simulink model "Wing_Aero"  (R2023b)
settings: Solver=ode3  StartTime=0.0  StopTime=1  FixedStep=0.01  RelTol=1e-3
undefined symbols (not defined in the file): alpha_C_d, alpha_C_l, b_Wing_Half, c, C_d, C_l, dr, l_Wing, num_Blade, r, thickness_Wing, throttle, V
libraries: spsMeanLib x7, simulink_extras x2, matrix_library x1
settings Model: Creator=iwl  LastModifiedBy=iwl

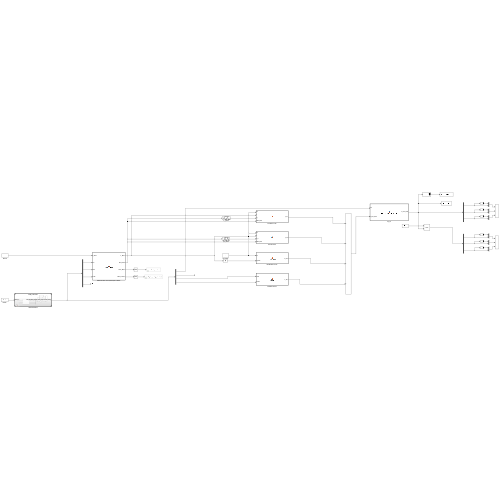
[thumbnail: Simulink's stored preview of the top-level diagram]
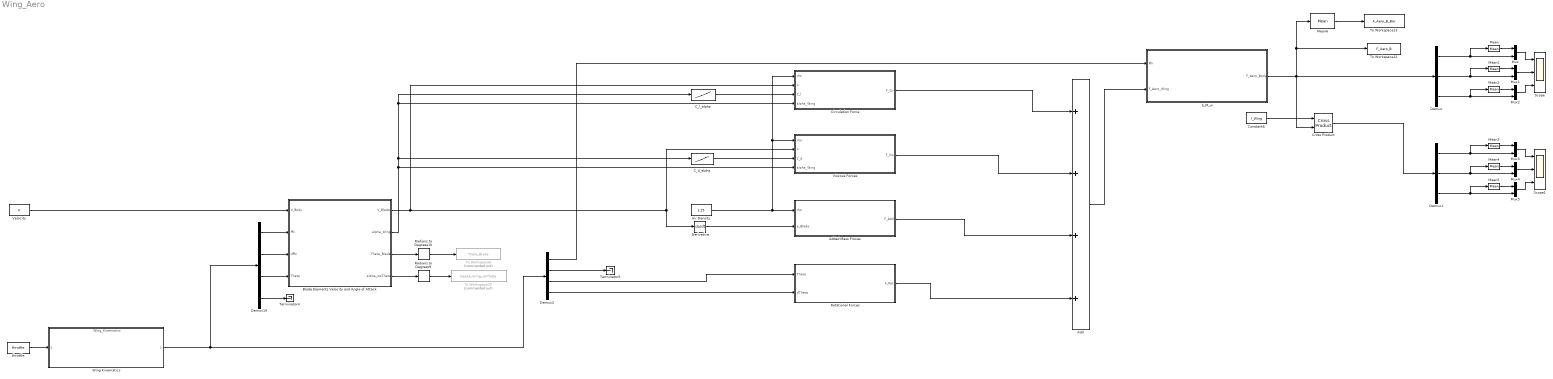
== system Wing_Aero ==
  Add : Sum  Inputs=++++
  Added Mass Froces : MATLAB Function  TreatAsAtomicUnit=on
  Air Density : Constant  Value=1.25
  Blade Elements Velocity and Angle of Attack : MATLAB Function  TreatAsAtomicUnit=on
  C_d_alpha : Lookup_n-D  NumberOfTableDimensions=1  BreakpointsForDimension1=alpha_C_d  Table=C_d  InternalRulePriority=Speed  RndMeth=Simplest
  C_l_alpha : Lookup_n-D  NumberOfTableDimensions=1  BreakpointsForDimension1=alpha_C_l  Table=C_l  InternalRulePriority=Speed  RndMeth=Simplest
  Circulation Force : MATLAB Function  TreatAsAtomicUnit=on
  Constant6 : Constant  Value=l_Wing
  Cross Product : matrix_library/Cross Product
  Demux : Demux  Outputs=3
  Demux1 : Demux  Outputs=3
  Demux19 : Demux
  Demux2 : Demux
  Derivative : Derivative
  Mean{,1..6} (7 alike) : spsMeanLib/Mean  Freq=f_max  Vinit=0  Ts=0
  Mux{,1..5} (6 alike) : Mux  Inputs=2
  Radians to Degrees10 : simulink_extras/Transformations/Radians to Degrees
  Radians to Degrees9 : simulink_extras/Transformations/Radians to Degrees
  Rotational Forces : MATLAB Function  TreatAsAtomicUnit=on
  Scope : Scope  NumInputPorts=3
  Scope1 : Scope  NumInputPorts=3
  Terminator4 : Terminator
  Terminator5 : Terminator
  To Workspace12 : ToWorkspace  VariableName=F_Aero_B  SampleTime=-1
  To Workspace13 : ToWorkspace  VariableName=F_Aero_B_Bar  SampleTime=-1
  To Workspace23 : ToWorkspace  Commented=on  VariableName=alapha_Wing_woTheta  SampleTime=-1
  To Workspace6 : ToWorkspace  Commented=on  VariableName=Theta_Blade  SampleTime=-1
  Velocity : Constant  Value=V
  Viscous Forces : MATLAB Function  TreatAsAtomicUnit=on
  Wing Kinematics : ModelReference  ModelNameDialog=Wing_Kinematics.slx  SimulationMode=Normal  ModelReferenceVersion=4.4
  b_M_w : MATLAB Function  TreatAsAtomicUnit=on
  throttle : Constant  Value=throttle
  wires:
  Demux19/4 -> Terminator4/1
  Radians to Degrees9/1 -> To Workspace23/1
  Demux2/2 -> Terminator5/1
  Demux19/1 -> Blade Elements Velocity and Angle of Attack/2(Phi)
  Blade Elements Velocity and Angle of Attack/3(Theta_Blade) -> Radians to Degrees10/1
  throttle/1 -> Wing Kinematics/1
  Demux19/2 -> Blade Elements Velocity and Angle of Attack/3(dPhi)
  Demux19/3 -> Blade Elements Velocity and Angle of Attack/4(Theta)
  Radians to Degrees10/1 -> To Workspace6/1
  Blade Elements Velocity and Angle of Attack/4(alpha_woTheta) -> Radians to Degrees9/1
  Wing Kinematics/1 -> Demux2/1, Demux19/1
  b_M_w/1(F_Aero_Body) -> Cross Product/2, Demux/1, Mean6/1, To Workspace12/1
  Add/1 -> b_M_w/2(F_Aero_Wing)
  Demux2/4 -> Rotational Forces/2(dTheta)
  Added Mass Froces/1(F_Add) -> Add/3
  Derivative/1 -> Added Mass Froces/2(a_Blade)
  Blade Elements Velocity and Angle of Attack/2(alpha_Wing) -> Circulation Force/4(alpha_Wing), C_l_alpha/1, C_d_alpha/1, Viscous Forces/4(alpha_Wing)
  C_l_alpha/1 -> Circulation Force/3(C_l)
  Circulation Force/1(F_Cir) -> Add/1
  Air Density/1 -> Circulation Force/1(rho), Viscous Forces/1(rho), Added Mass Froces/1(rho)
  Rotational Forces/1(F_Rot) -> Add/4
  Viscous Forces/1(F_Vis) -> Add/2
  C_d_alpha/1 -> Viscous Forces/3(C_d)
  Blade Elements Velocity and Angle of Attack/1(V_Blade) -> Viscous Forces/2(V), Derivative/1, Circulation Force/2(V)
  Constant6/1 -> Cross Product/1
  Demux2/1 -> b_M_w/1(Phi)
  Mean6/1 -> To Workspace13/1
  Demux2/3 -> Rotational Forces/1(Theta)
  Velocity/1 -> Blade Elements Velocity and Angle of Attack/1(V_Body)
  Demux/2 -> Mean1/1, Mux1/2
  Demux/1 -> Mux/2, Mean/1
  Demux/3 -> Mean2/1, Mux2/2
  Mean/1 -> Mux/1
  Mux/1 -> Scope/1
  Mean1/1 -> Mux1/1
  Mux1/1 -> Scope/2
  Mean2/1 -> Mux2/1
  Mux2/1 -> Scope/3
  Demux1/1 -> Mux3/2, Mean3/1
  Mux5/1 -> Scope1/3
  Cross Product/1 -> Demux1/1
  Mean3/1 -> Mux3/1
  Mux4/1 -> Scope1/2
  Demux1/2 -> Mean4/1, Mux4/2
  Mean4/1 -> Mux4/1
  Demux1/3 -> Mean5/1, Mux5/2
  Mean5/1 -> Mux5/1
  Mux3/1 -> Scope1/1

== matlab function Wing_Aero/Blade Elements Velocity and Angle of Attack ==
  data: V_Body input; Phi input; dPhi input; Theta input; V_Blade output; alpha_Wing output; Theta_Blade output; alpha_woTheta output; r parameter; b_Wing_Half parameter
function [V_Blade, alpha_Wing, Theta_Blade, alpha_woTheta] = V_alpha_Wing(V_Body, Phi, dPhi, Theta, r, b_Wing_Half)

    %% in local wing frame
    V_Flapping = r* dPhi .* [0; 0; 1];
    V_Body_W = [1 0 0; 0 cos(Phi) sin(Phi); 0 -sin(Phi) cos(Phi)] * V_Body;
    V_Blade = [V_Body_W(1); 0; V_Body_W(3)] + V_Flapping;

    %% in body frame
    % V_Flapping = r* dPhi .* [0; 0; cos(Phi)];
    % V_Total = [V(1); 0; V(3)] + V_Flapping;
    
    %% aoa
    Theta_Blade = Theta * r / b_Wing_Half;

    alpha_Wing = atan2(V_Blade(3,:), V_Blade(1,:)) + Theta_Blade;
    alpha_woTheta = atan2(V_Blade(3,:), V_Blade(1,:));
    % alpha_Tail = alpha_mount + atan2(V_Body(3), V_Body(1));

end

== matlab function Wing_Aero/Circulation Force ==
  data: F_Cir output; rho input; V input; C_l input; alpha_Wing input; c parameter; dr parameter
function F_Cir = Circulation(rho, V, C_l, alpha_Wing, c, dr)
    
    % forces on each blade element in WING frame
    dF_Cir = sum(0.5 * rho * V .* V .* C_l .* c * dr) .* [sin(alpha_Wing); zeros(1, size(alpha_Wing, 2)); -cos(alpha_Wing)];

    % dM_Circ = corss(l, dF_Circ);

    F_Cir = 2* sum(dF_Cir, 2);

    % M_Circ = 2 * sum(dM_Circ, 2);
    
end

== matlab function Wing_Aero/Added Mass Froces ==
  data: rho input; a_Blade input; num_Blade parameter; c parameter; F_Add output; thickness_Wing parameter; dr parameter
function F_Add  = Added_Mass(rho, a_Blade, num_Blade, c, thickness_Wing, dr)

    m_11 = 0.25* pi* rho* thickness_Wing^2 * ones(size(c));
    m_22 = 0.25* pi* rho* c.^2;

    dF_Add = -[m_11.* a_Blade(1,:); zeros(1, num_Blade); m_22.* a_Blade(3,:)].* dr;
    F_Add = 2* sum(dF_Add, 2);
        
end

== matlab function Wing_Aero/Rotational Forces ==
  data: Theta input; F_Rot output; dTheta input; c parameter; dr parameter
function F_Rot = Rotational(Theta, dTheta, c, dr)
    
    % c_R = 0.1666 - 0.374
    c_R = 0.1666;

    dF_Rot = c_R * dTheta .* c .* c * dr .* [cos(Theta); 0 ; sin(Theta)];
    
    F_Rot = 2* sum(dF_Rot, 2);

end

== matlab function Wing_Aero/b_M_w ==
  data: Phi input; F_Aero_Wing input; F_Aero_Body output
function F_Aero_Body = Transformation_Wing_to_Body(Phi, F_Aero_Wing)
    
    F_Aero_Body = [1 0 0; 0 cos(Phi) -sin(Phi); 0 sin(Phi) cos(Phi)] * F_Aero_Wing;

    F_Aero_Body(2) = 0;
    
end

== matlab function Wing_Aero/Viscous Forces ==
  data: rho input; F_Vis output; V input; C_d input; alpha_Wing input; c parameter; dr parameter
function F_Vis   = Viscous(rho, V, C_d, alpha_Wing, c, dr)
       
    dF_Vis = sum(0.5 * rho * V .* V .* C_d .* c * dr) .* [-cos(alpha_Wing); zeros(1, size(alpha_Wing, 2)); -sin(alpha_Wing)];

    F_Vis = 2* sum(dF_Vis, 2);
    
end
